simulink model "sim_linear_stateObserver_2017a"  (R2017a)
settings: Solver=ode4  StartTime=0.0  StopTime=inf  FixedStep=0.01  RelTol=1e-3
InitFcn:
  | run('initialize_system.m')
values from neighbouring files (symbols this model uses):
  Ac = [d_f1_dth,d_f1_dyw,d_f1_dw_th,d_f1_dw_yw ... (first row only)    [linearize_heli.m]
  Bc = [d_f1_Vmp,d_f1_Vmy ... (first row only)    [linearize_heli.m]
  Cc = [1,0,0,0;0,1,0,0]    [linearize_heli.m]
  th_op = -30*pi/180    (= -0.523598775598)    [initialize_system.m]
  Vmp_op = (Kyy*m_heli*g*cos(th_op)*l_cm) / (Kyy*Kpp - Kyp*Kpy)    [initialize_system.m]
  Vmy_op = (Kyp*Vmp_op) / (Kyy)    [initialize_system.m]
  w_th_op = 0    [initialize_system.m]
  w_yw_op = 0    [initialize_system.m]
  yw_op = pi/2    (= 1.57079632679)    [initialize_system.m]
undefined symbols (not defined in the file or in its folder): L
libraries: realtime_pacer_lib x1
settings Model: Creator=engen  LastModifiedBy=ronni
settings DataIOCC: ReturnWorkspaceOutputs=on
settings SFSimCC: SimUseLocalCustomCode=on
settings RTWCC: RTWUseLocalCustomCode=on

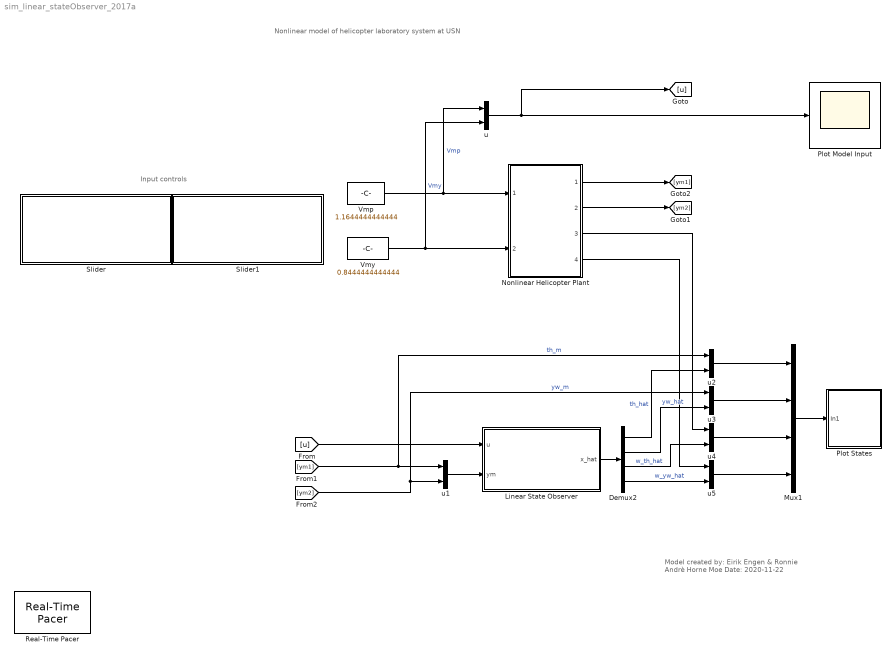
== system sim_linear_stateObserver_2017a ==
  note: Input controls
  note: Model created by:
      | Eirik Engen & Ronnie Andrè Horne Moe
      | Date: 2020-11-22
  note: Nonlinear model of helicopter laboratory system at USN
  Demux2 : Demux
  Linear State Observer : Subsystem
  Mux1 : Mux
  Nonlinear Helicopter Plant : ModelReference  ModelNameDialog=Nonlinear_Helicopter_Plant  ModelReferenceVersion=1.161  CopyOfModelProtected=on
  Plot Model Input : Scope
  Plot States : Subsystem
  Real-Time Pacer : realtime_pacer_lib/Real-Time Pacer  simTimePerRealTime=1
  Slider : Subsystem  DialogController=hmiCreateDDGDialog  IsWebBlock=on  mask(MWDashboardBlock){webBlockId=2715f4dd-60c0-4828-bf7c-a0e905dab087, webBlockType=slider, ShowInLibBrowser=on, ShowInitialText=on, HMISrcModelName=sim_linear_stateObserver_2017a}
      mask prompts: webBlockId "WebBlock Id"; webBlockType "WebBlock Type"; HMISrcModelName "Source Model"
      mask help: Set value to tune parameters or variables.
      mask Help: helpview([docroot '/mapfiles/simulink.map'], 'hmi_slider')
      mask Display:
      | if strcmp(get_param(bdroot(gcb),'BlockDiagramType'),'library')
      |  image([(matlabroot) '/toolbox/simulink/hmi/icons/Slider.png'])
      | end
  Slider1 : Subsystem  DialogController=hmiCreateDDGDialog  IsWebBlock=on  mask(MWDashboardBlock){webBlockId=f4af4151-69d5-4f46-932c-62e191981466, webBlockType=slider, ShowInLibBrowser=on, ShowInitialText=on, HMISrcModelName=sim_linear_stateObserver_2017a}
      mask prompts: webBlockId "WebBlock Id"; webBlockType "WebBlock Type"; HMISrcModelName "Source Model"
      mask help: Set value to tune parameters or variables.
      mask Help: helpview([docroot '/mapfiles/simulink.map'], 'hmi_slider')
      mask Display:
      | if strcmp(get_param(bdroot(gcb),'BlockDiagramType'),'library')
      |  image([(matlabroot) '/toolbox/simulink/hmi/icons/Slider.png'])
      | end
  Vmp : Constant  Value=1.1644444444444  SampleTime=-1
  Vmy : Constant  Value=0.8444444444444  SampleTime=-1
  u{,1..5} (6 alike) : Mux  Inputs=2
  wires:
  Vmp/1 -> u/1, Nonlinear Helicopter Plant/1  "Vmp"
  Vmy/1 -> u/2, Nonlinear Helicopter Plant/2  "Vmy"
  Nonlinear Helicopter Plant/1 -> [ym1]
  Nonlinear Helicopter Plant/2 -> [ym2]
  Nonlinear Helicopter Plant/3 -> u4/1
  Nonlinear Helicopter Plant/4 -> u5/1
  u/1 -> [u], Plot Model Input/1
  [u] -> Linear State Observer/1(u)
  u1/1 -> Linear State Observer/2(ym)
  Linear State Observer/1(x_hat) -> Demux2/1
  Mux1/1 -> Plot States/1(In1)
  u2/1 -> Mux1/1
  u3/1 -> Mux1/2
  Demux2/1 -> u2/2  "th_hat"
  Demux2/2 -> u3/2  "yw_hat"
  u5/1 -> Mux1/4
  u4/1 -> Mux1/3
  [ym1] -> u2/1, u1/1  "th_m"
  Demux2/4 -> u5/2  "w_yw_hat"
  Demux2/3 -> u4/2  "w_th_hat"
  [ym2] -> u3/1, u1/2  "yw_m"

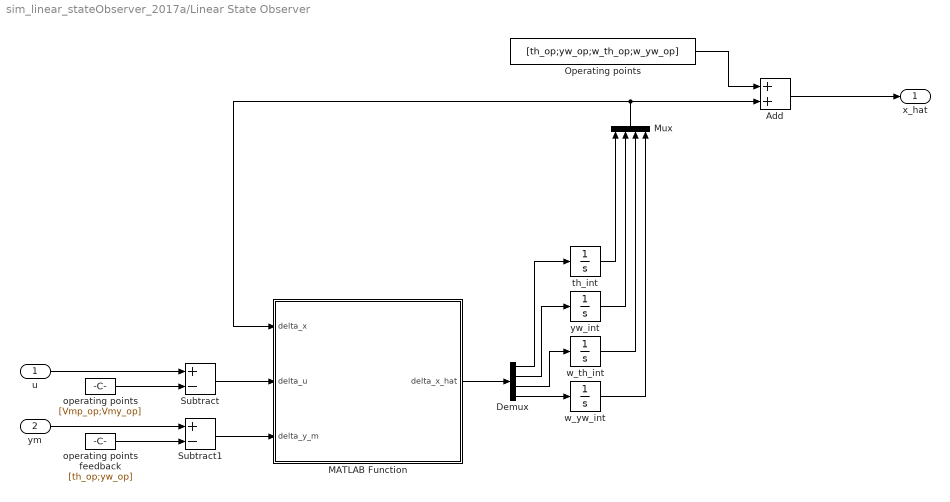
== system sim_linear_stateObserver_2017a/Linear State Observer ==
  u : Inport
  ym : Inport  Port=2
  Add : Sum
  Demux : Demux
  MATLAB Function : MATLAB Function  TreatAsAtomicUnit=on
  Mux : Mux
  Operating points : Constant  Value=[th_op;yw_op;w_th_op;w_yw_op]
  Subtract : Sum  Inputs=+-
  Subtract1 : Sum  Inputs=+-
  operating points : Constant  Value=[Vmp_op;Vmy_op]
  operating points feedback : Constant  Value=[th_op;yw_op]
  th_int : Integrator
  w_th_int : Integrator
  w_yw_int : Integrator
  yw_int : Integrator
  x_hat : Outport
  wires:
  MATLAB Function/1(delta_x_hat) -> Demux/1
  u/1 -> Subtract/1
  operating points/1 -> Subtract/2
  Subtract/1 -> MATLAB Function/2(delta_u)
  Mux/1 -> MATLAB Function/1(delta_x), Add/2
  Demux/1 -> th_int/1
  Demux/2 -> yw_int/1
  Demux/3 -> w_th_int/1
  Demux/4 -> w_yw_int/1
  th_int/1 -> Mux/1
  yw_int/1 -> Mux/2
  w_th_int/1 -> Mux/3
  w_yw_int/1 -> Mux/4
  Subtract1/1 -> MATLAB Function/3(delta_y_m)
  ym/1 -> Subtract1/1
  operating points feedback/1 -> Subtract1/2
  Operating points/1 -> Add/1
  Add/1 -> x_hat/1

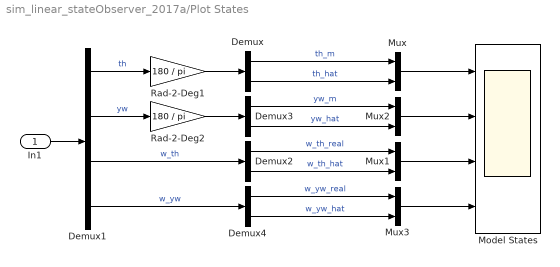
== system sim_linear_stateObserver_2017a/Plot States ==
  In1 : Inport
  Demux{,2..4} (4 alike) : Demux  Outputs=2
  Demux1 : Demux
  Model States : Scope  NumInputPorts=4
  Mux{,1..3} (4 alike) : Mux  Inputs=2
  Rad-2-Deg1 : Gain  Gain=180 / pi
  Rad-2-Deg2 : Gain  Gain=180 / pi
  wires:
  In1/1 -> Demux1/1
  Demux/1 -> Mux/1  "th_m"
  Demux/2 -> Mux/2  "th_hat"
  Demux3/1 -> Mux2/1  "yw_m"
  Demux3/2 -> Mux2/2  "yw_hat"
  Demux2/1 -> Mux1/1  "w_th_real"
  Demux2/2 -> Mux1/2  "w_th_hat"
  Demux4/1 -> Mux3/1  "w_yw_real"
  Demux4/2 -> Mux3/2  "w_yw_hat"
  Demux1/1 -> Rad-2-Deg1/1  "th"
  Demux1/2 -> Rad-2-Deg2/1  "yw"
  Demux1/3 -> Demux2/1  "w_th"
  Demux1/4 -> Demux4/1  "w_yw"
  Mux/1 -> Model States/1
  Mux2/1 -> Model States/2
  Mux1/1 -> Model States/3
  Mux3/1 -> Model States/4
  Rad-2-Deg2/1 -> Demux3/1
  Rad-2-Deg1/1 -> Demux/1

== system sim_linear_stateObserver_2017a/Slider ==

== system sim_linear_stateObserver_2017a/Slider1 ==

== matlab function sim_linear_stateObserver_2017a/Linear State Observer/MATLAB Function ==
  data: delta_x input; delta_u input; delta_x_hat output size=4; delta_y_m input; Ac parameter; Bc parameter; Cc parameter; L parameter
function delta_x_hat = linear_state_observer(delta_x, delta_u,delta_y_m,Ac,Bc,Cc,L)
    %apriori state
    delta_x_hat = Ac*delta_x + Bc*delta_u;
    %estimated output    
    y_hat = Cc*delta_x;
    % aposteriori state
    delta_x_hat = delta_x_hat + L*(delta_y_m - y_hat);
